simulink model "Project_sim"  (R2016b)
settings: Solver=FixedStepAuto  StartTime=0.0  StopTime=1  FixedStep=.02  RelTol=1e-3
libraries: simulink x1
settings Model: Creator=hp  LastModifiedBy=hp

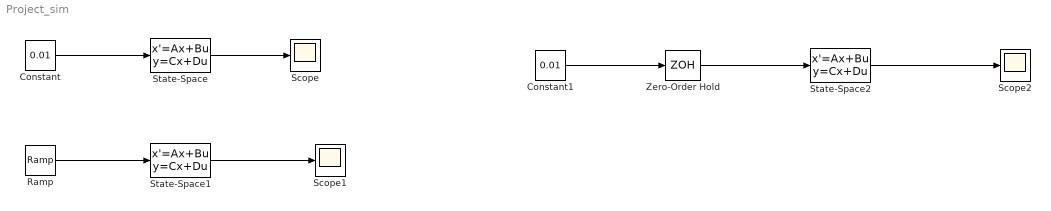
== system Project_sim ==
  Constant : Constant  Description=Simulation Model Input  Value=0.01  SampleTime=1
      settings: AttributesFormatString=|
      | Simulation Model
      | Input-Constant
  Constant1 : Constant  Description=Simulation Model Input  Value=0.01  SampleTime=1
      settings: AttributesFormatString=|
      | Simulation Model
      | Input-Constant
  Ramp : simulink/Sources/Ramp  Description=|  slope=.001  start=0  X0=0
      | Simulation Model
      | Input-Linear variable
      settings: AttributesFormatString=|
      | Simulation Model
      | Input-Linear
  Scope : Scope
      settings: Description=Output for constant Input
      settings: AttributesFormatString=|
      | Output
      | constant Input
  Scope1 : Scope
      settings: Description=Output for Linear Input
      settings: AttributesFormatString=|
      | Output
      |  Linear Input
      settings: ClipboardFcn=|
      | Output
      | Linear Input
  Scope2 : Scope
      settings: Description=Output for constant Input
      settings: AttributesFormatString=|
      | Output ZOH
      | constant Input
  State-Space : StateSpace  Tag=Ballbot  Description=|  A=|  B=|  C=[1, 0, 0, 0; 0, 0, 1, 0]  D=[0; 0]  X0=0
      A=|
      | [ 0, 1.0000, 0, 0; 0, -0.6698, -477.3945, 0; 0, 0, 0, 1.0000;
      | 0, 0.1477,  122.6790, 0]
      B=|
      | [0;
      | 69.7518;
      | 0;
      | -15.2579]
      Description=|
      | State space representation of Ballbot
      | Constant Input
      settings: AttributesFormatString=|
      | State space representation of Ballbot
      | Constant Input
  State-Space1 : StateSpace  Tag=Ballbot  Description=|  A=|  B=|  C=[1, 0, 0, 0; 0, 0, 1, 0]  D=[0; 0]  X0=0
      A=|
      | [ 0, 1.0000, 0, 0; 0, -0.6698, -477.3945, 0; 0, 0, 0, 1.0000;
      | 0, 0.1477,  122.6790, 0]
      B=|
      | [0;
      | 69.7518;
      | 0;
      | -15.2579]
      Description=|
      | State space representation of Ballbot
      | Linear Input
      settings: AttributesFormatString=|
      | State space representation of Ballbot
      | Linear Input
  State-Space2 : StateSpace  Tag=Ballbot  Description=|  A=|  B=|  C=[1, 0, 0, 0; 0, 0, 1, 0]  D=[0; 0]  X0=0
      A=|
      | [ 0, 1.0000, 0, 0; 0, -0.6698, -477.3945, 0; 0, 0, 0, 1.0000;
      | 0, 0.1477,  122.6790, 0]
      B=|
      | [0;
      | 69.7518;
      | 0;
      | -15.2579]
      Description=|
      | State space representation of Ballbot
      | Linear Input
      settings: AttributesFormatString=|
      | State space representation of Ballbot
      | Linear Input
  Zero-Order Hold : ZeroOrderHold  SampleTime=.005
  wires:
  Constant/1 -> State-Space/1
  State-Space/1 -> Scope/1
  State-Space1/1 -> Scope1/1
  Ramp/1 -> State-Space1/1
  Constant1/1 -> Zero-Order Hold/1
  Zero-Order Hold/1 -> State-Space2/1
  State-Space2/1 -> Scope2/1
